simulink model "modello_nonlineare_carroponte"  (R2018b)
settings: Solver=VariableStepAuto  StartTime=0.0  StopTime=10.0  RelTol=1e-3
values from neighbouring files (symbols this model uses):
  alpha_0 = pi/2    (= 1.57079632679)    [Script_inizializzazione_carroponte.m]
  alpha_dot_0 = 0    [Script_inizializzazione_carroponte.m]
  cc = 5e3    (= 5000)    [Script_inizializzazione_carroponte.m]
  cm = 100    [Script_inizializzazione_carroponte.m]
  g = 9.81    [Script_inizializzazione_carroponte.m]
  L = 2.5    [Script_inizializzazione_carroponte.m]
  mc = 300    [Script_inizializzazione_carroponte.m]
  mm = 1000    [Script_inizializzazione_carroponte.m]
  xc_0 = 0    [Script_inizializzazione_carroponte.m]
  xc_dot_0 = 0    [Script_inizializzazione_carroponte.m]
settings Model: Creator=franc  LastModifiedBy=franc

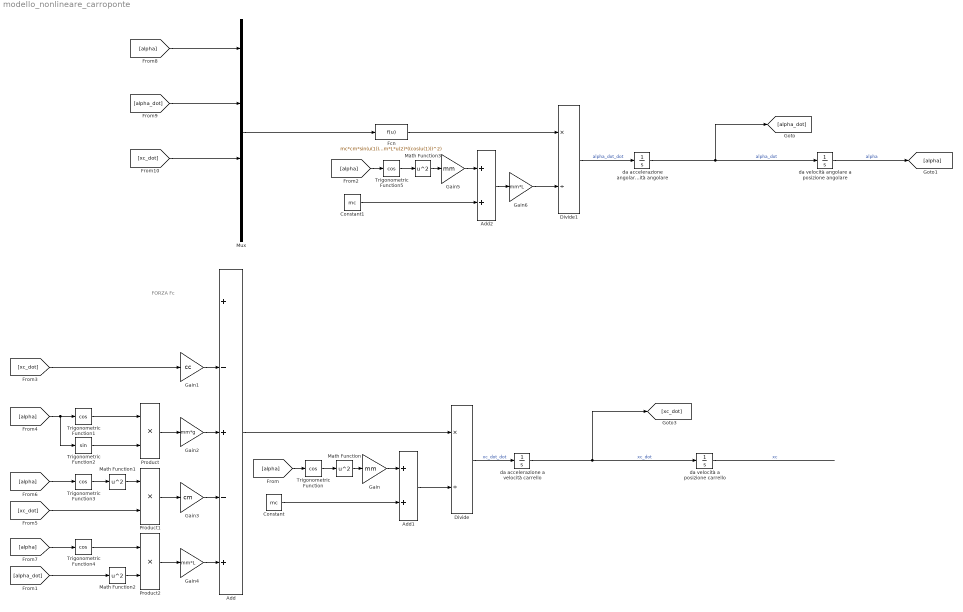
== system modello_nonlineare_carroponte ==
  note: FORZA Fc
  Add : Sum  Inputs=+-+-+
  Add1 : Sum
  Add2 : Sum
  Constant : Constant  Value=mc
  Constant1 : Constant  Value=mc
  Divide : Product  Inputs=*/
  Divide1 : Product  Inputs=*/
  "Fcn " : Fcn  Expr=mc*cm*sin(u(1))*u(3) - mm*cc*sin(u(1))*u(3) + (mm^2)*L*sin(u(1))*cos(u(1))*(u(2)^2) + mm*sin(u(1))*u(4) + (mm^2)*g*cos(u(1)) + mc*mm*g*cos(u(1)) - mc*cm*L*u(2) - mm*cm*L*u(2)*((cos(u(1)))^2)
  Gain : Gain  Gain=mm
  Gain1 : Gain  Gain=cc
  Gain2 : Gain  Gain=mm*g
  Gain3 : Gain  Gain=cm
  Gain4 : Gain  Gain=mm*L
  Gain5 : Gain  Gain=mm
  Gain6 : Gain  Gain=mm*L
  Math Function{,1..3} (4 alike) : Math  Operator=square  SaturateOnIntegerOverflow=on
  Mux : Mux
  Product : Product
  Product1 : Product
  Product2 : Product
  Trigonometric Function{,1,3..5} (5 alike) : Trigonometry  Operator=cos
  Trigonometric Function2 : Trigonometry
  da accelerazione a velocità carrello : Integrator  InitialCondition=xc_dot_0
  da accelerazione angolare a velocità angolare : Integrator  InitialCondition=alpha_dot_0
  da velocità a posizione carrello : Integrator  InitialCondition=xc_0
  da velocità angolare a posizione angolare : Integrator  InitialCondition=alpha_0
  wires:
  [xc_dot] -> Mux/3
  da accelerazione angolare a velocità angolare/1 -> [alpha_dot], da velocità angolare a posizione angolare/1  "alpha_dot"
  "Fcn "/1 -> Divide1/1
  Mux/1 -> "Fcn "/1
  Product1/1 -> Gain3/1
  [alpha_dot] -> Math Function2/1
  [alpha] -> Trigonometric Function5/1
  Constant1/1 -> Add2/2
  [alpha] -> Trigonometric Function2/1, Trigonometric Function1/1
  [xc_dot] -> Product1/2
  Divide/1 -> da accelerazione a velocità carrello/1  "xc_dot_dot"
  Gain6/1 -> Divide1/2
  Divide1/1 -> da accelerazione angolare a velocità angolare/1  "alpha_dot_dot"
  Gain5/1 -> Add2/1
  Gain/1 -> Add1/1
  Math Function3/1 -> Gain5/1
  [alpha] -> Trigonometric Function/1
  [xc_dot] -> Gain1/1
  Trigonometric Function/1 -> Math Function/1
  Add2/1 -> Gain6/1
  [alpha_dot] -> Mux/2
  Math Function2/1 -> Product2/2
  da velocità angolare a posizione angolare/1 -> [alpha]  "alpha"
  da accelerazione a velocità carrello/1 -> da velocità a posizione carrello/1, [xc_dot]  "xc_dot"
  Product2/1 -> Gain4/1
  Add1/1 -> Divide/2
  Constant/1 -> Add1/2
  Gain1/1 -> Add/2
  [alpha] -> Mux/1
  Trigonometric Function5/1 -> Math Function3/1
  Math Function/1 -> Gain/1
  Trigonometric Function2/1 -> Product/2
  [alpha] -> Trigonometric Function4/1
  Gain3/1 -> Add/4
  Add/1 -> Divide/1
  Product/1 -> Gain2/1
  Math Function1/1 -> Product1/1
  [alpha] -> Trigonometric Function3/1
  Gain4/1 -> Add/5
  ? -> Mux/4, Add/1
  Trigonometric Function3/1 -> Math Function1/1
  Gain2/1 -> Add/3
  Trigonometric Function1/1 -> Product/1
  Trigonometric Function4/1 -> Product2/1
  da velocità a posizione carrello/1 -> ?  "xc"
